simulink model "Van1"  (R2024b)
settings: Solver=ode3  StartTime=0.0  StopTime=10  FixedStep=0.001  RelTol=1e-3
Description:
  | 不同TP
settings Model: PacingRate=1000  Creator=繁星  LastModifiedBy=14422
settings SolverCC: ShapePreserveControl=EnableAll  ZeroCrossAlgorithm=Adaptive
settings DataIOCC: ReturnWorkspaceOutputs=off
settings OptimizationCC: ReuseModelBlockBuffer=off
settings ModelReferenceCC: EnableRefExpFcnMdlSchedulingChecks=on
settings RTWCC: GPUComputeCapability=3.5

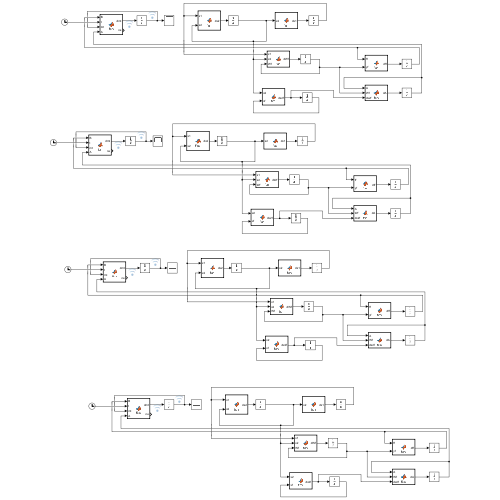
[thumbnail: Simulink's stored preview of the top-level diagram]
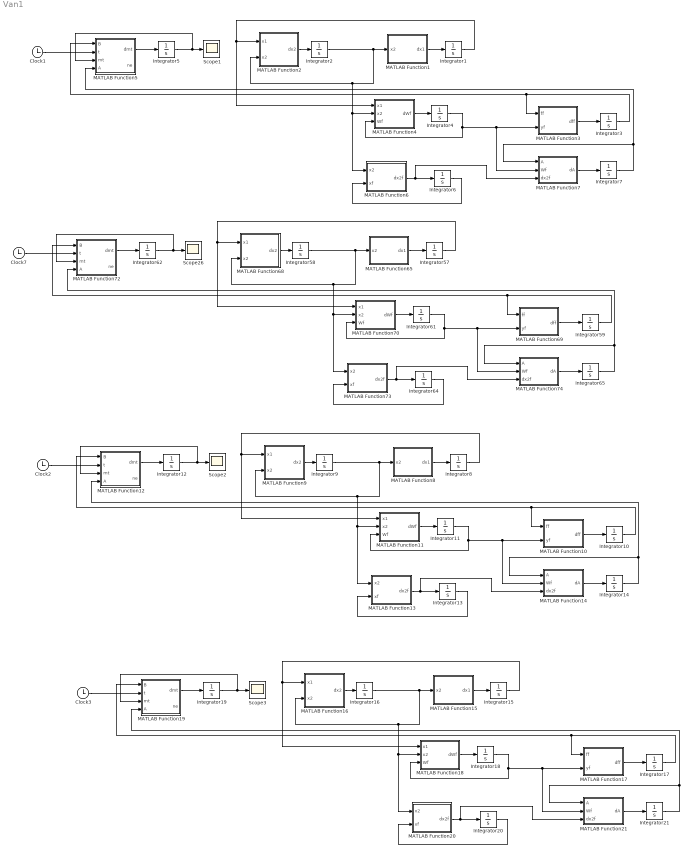
== system Van1 ==
  Clock{1..3,7} (4 alike) : Clock
  Integrator{1,8,15,57} (4 alike) : Integrator  InitialCondition=1
  Integrator{3,10,17,59} (4 alike) : Integrator  InitialCondition=[1 0 0;0 1 0;0 0 1]*1e-7
  Integrator{2,4..7,9,11..14,16,18..21,58,61..62,64..65} (20 alike) : Integrator
  MATLAB Function1 : MATLAB Function  TreatAsAtomicUnit=on
  MATLAB Function10 : MATLAB Function  TreatAsAtomicUnit=on
  MATLAB Function11 : MATLAB Function  TreatAsAtomicUnit=on
  MATLAB Function12 : MATLAB Function  TreatAsAtomicUnit=on
  MATLAB Function13 : MATLAB Function  TreatAsAtomicUnit=on
  MATLAB Function14 : MATLAB Function  TreatAsAtomicUnit=on
  MATLAB Function15 : MATLAB Function  TreatAsAtomicUnit=on
  MATLAB Function16 : MATLAB Function  TreatAsAtomicUnit=on
  MATLAB Function17 : MATLAB Function  TreatAsAtomicUnit=on
  MATLAB Function18 : MATLAB Function  TreatAsAtomicUnit=on
  MATLAB Function19 : MATLAB Function  TreatAsAtomicUnit=on
  MATLAB Function2 : MATLAB Function  TreatAsAtomicUnit=on
  MATLAB Function20 : MATLAB Function  TreatAsAtomicUnit=on
  MATLAB Function21 : MATLAB Function  TreatAsAtomicUnit=on
  MATLAB Function3 : MATLAB Function  TreatAsAtomicUnit=on
  MATLAB Function4 : MATLAB Function  TreatAsAtomicUnit=on
  MATLAB Function5 : MATLAB Function  TreatAsAtomicUnit=on
  MATLAB Function6 : MATLAB Function  TreatAsAtomicUnit=on
  MATLAB Function65 : MATLAB Function  TreatAsAtomicUnit=on
  MATLAB Function68 : MATLAB Function  TreatAsAtomicUnit=on
  MATLAB Function69 : MATLAB Function  TreatAsAtomicUnit=on
  MATLAB Function7 : MATLAB Function  TreatAsAtomicUnit=on
  MATLAB Function70 : MATLAB Function  TreatAsAtomicUnit=on
  MATLAB Function72 : MATLAB Function  TreatAsAtomicUnit=on
  MATLAB Function73 : MATLAB Function  TreatAsAtomicUnit=on
  MATLAB Function74 : MATLAB Function  TreatAsAtomicUnit=on
  MATLAB Function8 : MATLAB Function  TreatAsAtomicUnit=on
  MATLAB Function9 : MATLAB Function  TreatAsAtomicUnit=on
  Scope{1..3,26} (4 alike) : Scope
  wires:
  MATLAB Function73/1(dx2f) -> MATLAB Function74/3(dx2f), Integrator64/1
  Integrator62/1 -> MATLAB Function72/3(mt), Scope26/1
  MATLAB Function69/1(dff) -> Integrator59/1
  Integrator59/1 -> MATLAB Function72/1(B), MATLAB Function69/1(ff)
  MATLAB Function68/1(dx2) -> Integrator58/1
  MATLAB Function70/1(dWf) -> Integrator61/1
  Integrator61/1 -> MATLAB Function70/3(Wf), MATLAB Function74/2(Wf), MATLAB Function69/2(yf)
  MATLAB Function74/1(dA) -> Integrator65/1
  Integrator65/1 -> MATLAB Function74/1(A), MATLAB Function72/4(A)
  MATLAB Function65/1(dx1) -> Integrator57/1
  Integrator64/1 -> MATLAB Function73/2(xf)
  MATLAB Function72/1(dmt) -> Integrator62/1
  Clock7/1 -> MATLAB Function72/2(t)
  Integrator58/1 -> MATLAB Function70/2(x2), MATLAB Function73/1(x2), MATLAB Function68/2(x2), MATLAB Function65/1(x2)
  Integrator57/1 -> MATLAB Function70/1(x1), MATLAB Function68/1(x1)
  MATLAB Function3/1(dff) -> Integrator3/1
  MATLAB Function6/1(dx2f) -> MATLAB Function7/3(dx2f), Integrator6/1
  Integrator2/1 -> MATLAB Function4/2(x2), MATLAB Function6/1(x2), MATLAB Function2/2(x2), MATLAB Function1/1(x2)
  Integrator6/1 -> MATLAB Function6/2(xf)
  MATLAB Function1/1(dx1) -> Integrator1/1
  Clock1/1 -> MATLAB Function5/2(t)
  MATLAB Function7/1(dA) -> Integrator7/1
  Integrator1/1 -> MATLAB Function4/1(x1), MATLAB Function2/1(x1)
  Integrator7/1 -> MATLAB Function7/1(A), MATLAB Function5/4(A)
  MATLAB Function4/1(dWf) -> Integrator4/1
  Integrator4/1 -> MATLAB Function4/3(Wf), MATLAB Function7/2(Wf), MATLAB Function3/2(yf)
  Integrator5/1 -> MATLAB Function5/3(mt), Scope1/1
  Integrator3/1 -> MATLAB Function5/1(B), MATLAB Function3/1(ff)
  MATLAB Function5/1(dmt) -> Integrator5/1
  MATLAB Function2/1(dx2) -> Integrator2/1
  MATLAB Function10/1(dff) -> Integrator10/1
  MATLAB Function13/1(dx2f) -> MATLAB Function14/3(dx2f), Integrator13/1
  Integrator9/1 -> MATLAB Function11/2(x2), MATLAB Function13/1(x2), MATLAB Function9/2(x2), MATLAB Function8/1(x2)
  Integrator13/1 -> MATLAB Function13/2(xf)
  MATLAB Function8/1(dx1) -> Integrator8/1
  Clock2/1 -> MATLAB Function12/2(t)
  MATLAB Function14/1(dA) -> Integrator14/1
  Integrator8/1 -> MATLAB Function11/1(x1), MATLAB Function9/1(x1)
  Integrator14/1 -> MATLAB Function14/1(A), MATLAB Function12/4(A)
  MATLAB Function11/1(dWf) -> Integrator11/1
  Integrator11/1 -> MATLAB Function11/3(Wf), MATLAB Function14/2(Wf), MATLAB Function10/2(yf)
  Integrator12/1 -> MATLAB Function12/3(mt), Scope2/1
  Integrator10/1 -> MATLAB Function12/1(B), MATLAB Function10/1(ff)
  MATLAB Function12/1(dmt) -> Integrator12/1
  MATLAB Function9/1(dx2) -> Integrator9/1
  MATLAB Function17/1(dff) -> Integrator17/1
  MATLAB Function20/1(dx2f) -> MATLAB Function21/3(dx2f), Integrator20/1
  Integrator16/1 -> MATLAB Function18/2(x2), MATLAB Function20/1(x2), MATLAB Function16/2(x2), MATLAB Function15/1(x2)
  Integrator20/1 -> MATLAB Function20/2(xf)
  MATLAB Function15/1(dx1) -> Integrator15/1
  Clock3/1 -> MATLAB Function19/2(t)
  MATLAB Function21/1(dA) -> Integrator21/1
  Integrator15/1 -> MATLAB Function18/1(x1), MATLAB Function16/1(x1)
  Integrator21/1 -> MATLAB Function21/1(A), MATLAB Function19/4(A)
  MATLAB Function18/1(dWf) -> Integrator18/1
  Integrator18/1 -> MATLAB Function18/3(Wf), MATLAB Function21/2(Wf), MATLAB Function17/2(yf)
  Integrator19/1 -> MATLAB Function19/3(mt), Scope3/1
  Integrator17/1 -> MATLAB Function19/1(B), MATLAB Function17/1(ff)
  MATLAB Function19/1(dmt) -> Integrator19/1
  MATLAB Function16/1(dx2) -> Integrator16/1

== matlab function Van1/MATLAB Function12 ==
  data: B input; dmt output size=3,1; t input; mt input; A input size=3,1; ne output
function [dmt,ne]    = fcn(B,t,mt,A)





theta=[0.5;-1;1];
k1=1e-7;
ne=norm(theta-mt);%Parameter estimation error norm
k=0.2;
ee=B\A-(1*eye(3)-k1*eye(3)*exp(-1*t)/B)*mt;

Tp=3;%predefined constant

%Parameter update law
dmt=exp(abs(ee).^k).*sign(ee).*abs(ee).^(1-k)/(k*Tp);

== matlab function Van1/MATLAB Function13 ==
  data: x2 input; xf input; dx2f output
function dx2f  = fcn(x2,xf)


dx2f=-0.1*xf+x2;

== matlab function Van1/MATLAB Function14 ==
  data: A input; dA output; Wf input; dx2f input
function dA  = fcn(A,Wf,dx2f)


dA=-1*A+Wf'*dx2f;

== matlab function Van1/MATLAB Function8 ==
  data: x2 input; dx1 output
function dx1 = fcn(x2)
dx1=x2;

== matlab function Van1/MATLAB Function9 ==
  data: x1 input; x2 input size=1; dx2 output size=1
function dx2  = fcn(x1,x2)


theta=[0.5;-1;1];

u=0;
dx2=[-x1,x2,-x1*x1*x2]*theta+u;

== matlab function Van1/MATLAB Function15 ==
  data: x2 input; dx1 output
function dx1 = fcn(x2)
dx1=x2;

== matlab function Van1/MATLAB Function16 ==
  data: x1 input; x2 input size=1; dx2 output size=1
function dx2  = fcn(x1,x2)


theta=[0.5;-1;1];

u=0;
dx2=[-x1,x2,-x1*x1*x2]*theta+u;

== matlab function Van1/MATLAB Function17 ==
  data: ff input; dff output; yf input
function dff = fcn(ff,yf)


dff=-1*ff+yf'*yf;

== matlab function Van1/MATLAB Function18 ==
  data: x1 input; dWf output; x2 input; Wf input
function dWf  = fcn(x1,x2,Wf)

A=[-x1,x2,-x1*x1*x2];
dWf=-0.1*Wf+A;

== matlab function Van1/MATLAB Function19 ==
  data: B input; dmt output size=3,1; t input; mt input; A input size=3,1; ne output
function [dmt,ne]    = fcn(B,t,mt,A)





theta=[0.5;-1;1];
k1=1e-7;
ne=norm(theta-mt);%Parameter estimation error norm
k=0.2;
ee=B\A-(1*eye(3)-k1*eye(3)*exp(-1*t)/B)*mt;

Tp=4;%predefined constant

%Parameter update law
dmt=exp(abs(ee).^k).*sign(ee).*abs(ee).^(1-k)/(k*Tp);

== matlab function Van1/MATLAB Function20 ==
  data: x2 input; xf input; dx2f output
function dx2f  = fcn(x2,xf)


dx2f=-0.1*xf+x2;

== matlab function Van1/MATLAB Function21 ==
  data: A input; dA output; Wf input; dx2f input
function dA  = fcn(A,Wf,dx2f)


dA=-1*A+Wf'*dx2f;

== matlab function Van1/MATLAB Function65 ==
  data: x2 input; dx1 output
function dx1 = fcn(x2)
dx1=x2;

== matlab function Van1/MATLAB Function68 ==
  data: x1 input; x2 input size=1; dx2 output size=1
function dx2  = fcn(x1,x2)


theta=[0.5;-1;1];

u=0;
dx2=[-x1,x2,-x1*x1*x2]*theta+u;

== matlab function Van1/MATLAB Function69 ==
  data: ff input; dff output; yf input
function dff = fcn(ff,yf)


dff=-1*ff+yf'*yf;

== matlab function Van1/MATLAB Function70 ==
  data: x1 input; dWf output; x2 input; Wf input
function dWf  = fcn(x1,x2,Wf)

A=[-x1,x2,-x1*x1*x2];
dWf=-0.1*Wf+A;

== matlab function Van1/MATLAB Function72 ==
  data: B input; dmt output size=3,1; t input; mt input; A input size=3,1; ne output
function [dmt,ne]    = fcn(B,t,mt,A)





theta=[0.5;-1;1];
k1=1e-7;
ne=norm(theta-mt);%Parameter estimation error norm
k=0.2;
ee=B\A-(1*eye(3)-k1*eye(3)*exp(-1*t)/B)*mt;

Tp=2;%predefined constant

%Parameter update law
dmt=exp(abs(ee).^k).*sign(ee).*abs(ee).^(1-k)/(k*Tp);

== matlab function Van1/MATLAB Function73 ==
  data: x2 input; xf input; dx2f output
function dx2f  = fcn(x2,xf)


dx2f=-0.1*xf+x2;

== matlab function Van1/MATLAB Function1 ==
  data: x2 input; dx1 output
function dx1 = fcn(x2)
dx1=x2;

== matlab function Van1/MATLAB Function74 ==
  data: A input; dA output; Wf input; dx2f input
function dA  = fcn(A,Wf,dx2f)


dA=-1*A+Wf'*dx2f;

== matlab function Van1/MATLAB Function2 ==
  data: x1 input; x2 input size=1; dx2 output size=1
function dx2  = fcn(x1,x2)


theta=[0.5;-1;1];

u=0;
dx2=[-x1,x2,-x1*x1*x2]*theta+u;

== matlab function Van1/MATLAB Function3 ==
  data: ff input; dff output; yf input
function dff = fcn(ff,yf)


dff=-1*ff+yf'*yf;

== matlab function Van1/MATLAB Function4 ==
  data: x1 input; dWf output; x2 input; Wf input
function dWf  = fcn(x1,x2,Wf)

A=[-x1,x2,-x1*x1*x2];
dWf=-0.1*Wf+A;

== matlab function Van1/MATLAB Function5 ==
  data: B input; dmt output size=3,1; t input; mt input; A input size=3,1; ne output
function [dmt,ne]    = fcn(B,t,mt,A)





theta=[0.5;-1;1];
k1=1e-7;
ne=norm(theta-mt);%Parameter estimation error norm
k=0.2;
ee=B\A-(1*eye(3)-k1*eye(3)*exp(-1*t)/B)*mt;

Tp=1;%predefined constant

%Parameter update law
dmt=exp(abs(ee).^k).*sign(ee).*abs(ee).^(1-k)/(k*Tp);

== matlab function Van1/MATLAB Function6 ==
  data: x2 input; xf input; dx2f output
function dx2f  = fcn(x2,xf)


dx2f=-0.1*xf+x2;

== matlab function Van1/MATLAB Function7 ==
  data: A input; dA output; Wf input; dx2f input
function dA  = fcn(A,Wf,dx2f)


dA=-1*A+Wf'*dx2f;

== matlab function Van1/MATLAB Function10 ==
  data: ff input; dff output; yf input
function dff = fcn(ff,yf)


dff=-1*ff+yf'*yf;

== matlab function Van1/MATLAB Function11 ==
  data: x1 input; dWf output; x2 input; Wf input
function dWf  = fcn(x1,x2,Wf)

A=[-x1,x2,-x1*x1*x2];
dWf=-0.1*Wf+A;
